simulink model "EReg_Tank_Drain"  (R2025b)
settings: Solver=ode1  StartTime=0.0  StopTime=12  FixedStep=0.001  RelTol=1e-3
values from neighbouring files (symbols this model uses):
  A_3 = 13.27e-6    (= 1.327e-05)    [EReg_N2O_Simulink_Init.m]    (also in EReg_Tank_Drain_Init.m = 6e-05)
  Cd_3 = 0.6    [EReg_N2O_Simulink_Init.m]    (also in EReg_Tank_Drain_Init.m = 0.7)
  Feedforward = 0    [EReg_N2O_Simulink_Init.m]    (also in EReg_Tank_Drain_Init.m)
  hL_LUT = n2o_tab.h_L    [EReg_N2O_Simulink_Init.m]
  K_D = 3    [EReg_N2O_Simulink_Init.m]    (also in EReg_Tank_Drain_Init.m = 8; EReg_Tank_Drain_N2O_Sim.m = params.K_D)
  K_I = 15    [EReg_N2O_Simulink_Init.m]    (also in EReg_Tank_Drain_Init.m = 17; EReg_Tank_Drain_N2O_Sim.m = params.K_I)
  K_P = 20    [EReg_N2O_Simulink_Init.m]    (also in EReg_Tank_Drain_Init.m = 16; EReg_Tank_Drain_N2O_Sim.m = params.K_P)
  Kv_1_max = 1.5    [EReg_N2O_Simulink_Init.m]    (also in EReg_Tank_Drain_Init.m = 1; EReg_Tank_Drain_N2O_Sim.m = params.Kv_1_max)
  Kv_2 = 1    [EReg_Tank_Drain_Init.m]
  m_1_0 = rho_1_0 * V_1    (= 2.35097796073)    [EReg_N2O_Simulink_Init.m]    (also in EReg_Tank_Drain_Init.m = 2.2972972973; EReg_Tank_Drain_N2O_Sim.m = params.m_1_0)
  m_N2_ull_0 = rho_N2_init * V_ull_init    [EReg_N2O_Simulink_Init.m]
  m_N2O_liq_0 = 12    [EReg_N2O_Simulink_Init.m]
  P_1_0 = 300e5    (= 30000000)    [EReg_N2O_Simulink_Init.m]    (also in EReg_Tank_Drain_Init.m; EReg_Tank_Drain_N2O_Sim.m = params.P_1_0)
  P_atm = 25e5    (= 2500000)    [EReg_N2O_Simulink_Init.m]    (also in EReg_Tank_Drain_Init.m = 0; EReg_Tank_Drain_N2O_Sim.m = params.P_atm)
  P_sat_LUT = n2o_tab.P    [EReg_N2O_Simulink_Init.m]
  R_N2 = 296    [EReg_N2O_Simulink_Init.m]    (also in EReg_Tank_Drain_Init.m; EReg_Tank_Drain_N2O_Sim.m = params.R_N2)
  rho_1_0 = P_1_0 / (R_N2 * T_0_N2)    (= 345.732053049)    [EReg_N2O_Simulink_Init.m]    (also in EReg_Tank_Drain_Init.m = 337.837837838; EReg_Tank_Drain_N2O_Sim.m = m_1_0 / V_1)
  rhoL_LUT = n2o_tab.rho_L    [EReg_N2O_Simulink_Init.m]
  rhoV_LUT = n2o_tab.rho_V    [EReg_N2O_Simulink_Init.m]
  servo_off_setpoint = ones(1, Num_Steps)    [EReg_N2O_Simulink_Init.m]    (also in EReg_Tank_Drain_Init.m = zeros(1, Num_Steps))
  T_1_0 = T_0_N2    (= 293.15)    [EReg_N2O_Simulink_Init.m]    (also in EReg_Tank_Drain_N2O_Sim.m = P_1_0 / (rho_1_0 * R_N2))
  T_N2O_0 = T_0_N2    (= 293.15)    [EReg_N2O_Simulink_Init.m]
  T_sat_LUT = n2o_tab.T    [EReg_N2O_Simulink_Init.m]
  time = linspace(0, Sim_Duration, Num_Steps)    [EReg_N2O_Simulink_Init.m]    (also in EReg_Tank_Drain_Init.m; EReg_Tank_Drain_N2O_Sim.m = (0 : dt : t_end)')
  U_N2O_0 = m_N2O_liq_0 * uL_init + m_N2O_vap_init * uV_init    [EReg_N2O_Simulink_Init.m]
  uL_LUT = n2o_tab.u_L    [EReg_N2O_Simulink_Init.m]
  uV_LUT = n2o_tab.u_V    [EReg_N2O_Simulink_Init.m]
  V_1 = 6.8e-3    (= 0.0068)    [EReg_N2O_Simulink_Init.m]    (also in EReg_Tank_Drain_Init.m; EReg_Tank_Drain_N2O_Sim.m = params.V_1)
  V_2 = 30e-3    (= 0.03)    [EReg_N2O_Simulink_Init.m]    (also in EReg_Tank_Drain_Init.m = 0.025; EReg_Tank_Drain_N2O_Sim.m = params.V_2)
libraries: simulink x4, slpidlib x2
settings Model: Creator=marti  LastModifiedBy=Aziz
settings OptimizationCC: ReuseModelBlockBuffer=off
settings RTWCC: GPUComputeCapability=3.5

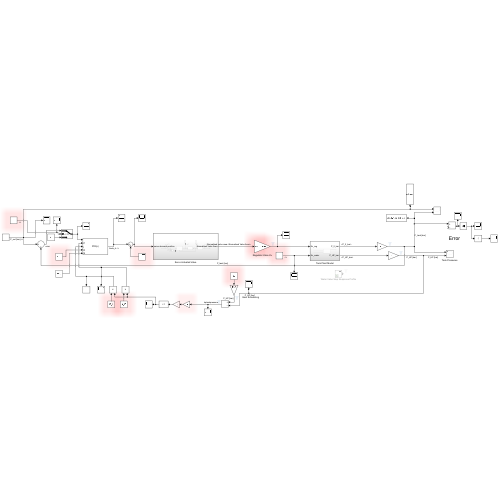
[thumbnail: Simulink's stored preview of the top-level diagram]
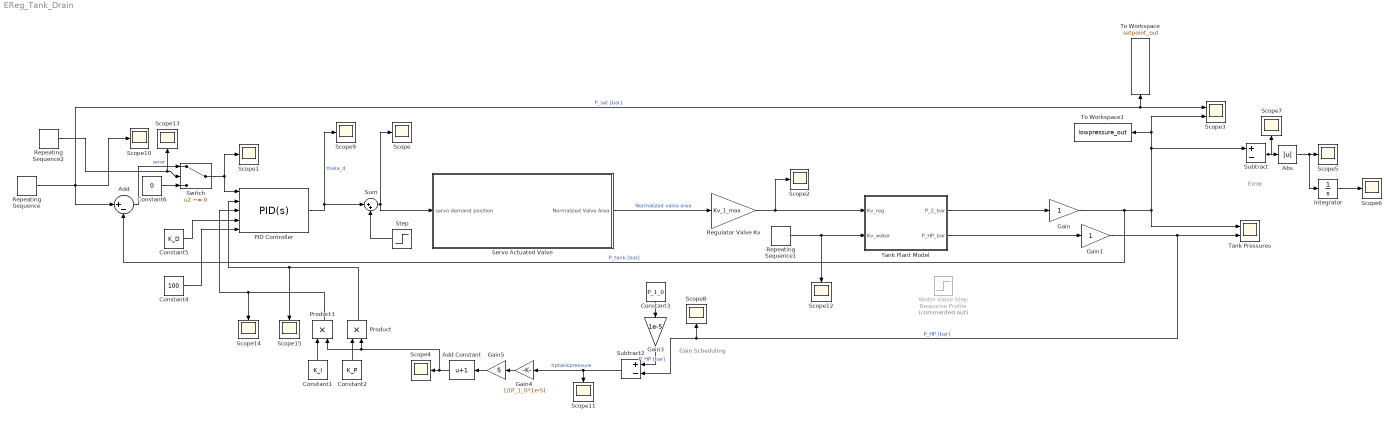
== system EReg_Tank_Drain ==
  note: Gain Scheduling
  note: Error
  Abs : Abs  SaturateOnIntegerOverflow=off
  Add : Sum  Inputs=|+-
  Add Constant : Bias  Bias=1  SaturateOnIntegerOverflow=off
  Constant1 : Constant  Value=K_I
  Constant2 : Constant  Value=K_P
  Constant3 : Constant  Value=P_1_0
  Constant4 : Constant  Value=100
  Constant5 : Constant  Value=K_D
  Constant6 : Constant  Value=0
  Gain : Gain
  Gain1 : Gain
  Gain3 : Gain  Gain=1e-5
  Gain4 : Gain  Gain=1/(P_1_0*1e-5)
  Gain5 : Gain  Gain=5
  Integrator : Integrator
  PID Controller : slpidlib/PID Controller  Controller=PID  Form=Parallel  TimeDomain=Continuous-time  UseExternalTs=off  SampleTime=-1  IntegratorMethod=Forward Euler  FilterMethod=Forward Euler  ControllerParametersSource=external  P=1.5  I=3  UseKiTs=off  D=0  UseExternalDerivativeSource=off  N=100  UseFilter=on  TunerSelectOption=Transfer Function Based (PID Tuner App)  InitialConditionSource=internal  InitialConditionForIntegrator=0  InitialConditionForFilter=0  DifferentiatorICPrevScaledInput=0  ExternalReset=none  TrackingMode=off  Kt=1  LimitOutput=off  SatLimitsSource=internal  UpperSaturationLimit=180  LowerSaturationLimit=0  LinearizeAsGain=on  AntiWindupMode=clamping  Kb=1  LimitIntegrator=on  UpperIntegratorSaturationLimit=20  LowerIntegratorSaturationLimit=-20  POutMin=[]  POutMax=[]  IOutMin=[]  IOutMax=[]  DOutMin=[]  DOutMax=[]  NOutMin=[]  NOutMax=[]  SumOutMin=[]  SumOutMax=[]  SaturationOutMin=[]  SaturationOutMax=[]  PParamMin=[]  PParamMax=[]  IParamMin=[]  IParamMax=[]  DParamMin=[]  DParamMax=[]  NParamMin=[]  NParamMax=[]  KbParamMin=[]  KbParamMax=[]  KtParamMin=[]  KtParamMax=[]  KbOutMin=[]  KbOutMax=[]  KtOutMin=[]  KtOutMax=[]  IntegratorOutMin=[]  IntegratorOutMax=[]  FilterOutMin=[]  FilterOutMax=[]  SumI1OutMin=[]  SumI1OutMax=[]  SumI2OutMin=[]  SumI2OutMax=[]  SumI3OutMin=[]  SumI3OutMax=[]  SumI4OutMin=[]  SumI4OutMax=[]  SumDOutMin=[]  SumDOutMax=[]  DifferentiatorOutMin=[]  DifferentiatorOutMax=[]  FilterDiffOutCoefMin=[]  FilterDiffOutCoefMax=[]  ReciprocalOutMin=[]  ReciprocalOutMax=[]  SumDenOutMin=[]  SumDenOutMax=[]  SumNumOutMin=[]  SumNumOutMax=[]  DivideOutMin=[]  DivideOutMax=[]  UdiffTsProdOutMin=[]  UdiffTsProdOutMax=[]  NTsProdOutMin=[]  NTsProdOutMax=[]  UintegralTsProdOutMin=[]  UintegralTsProdOutMax=[]  UngainTsProdOutMin=[]  UngainTsProdOutMax=[]  ClampingZeroOutDataTypeStr=Inherit: Inherit via back propagation  ClampingZeroOutMin=[]  ClampingZeroOutMax=[]  FilterDenConstantOutDataTypeStr=Inherit: Inherit via back propagation  FilterDenConstantOutMin=[]  FilterDenConstantOutMax=[]  PCopyOutDataTypeStr=Inherit: Inherit via back propagation  PCopyOutMin=[]  PCopyOutMax=[]  NCopyOutDataTypeStr=Inherit: Inherit via back propagation  NCopyOutMin=[]  NCopyOutMax=[]  IntegratorContinuousStateAttributes=''  IntegratorStateMustResolveToSignalObject=off  IntegratorRTWStateStorageClass=Auto  FilterContinuousStateAttributes=''  FilterStateMustResolveToSignalObject=off  FilterRTWStateStorageClass=Auto  ParallelPVariant=ExternalParameters  IdealPVariant=Disabled  IVariant=ExternalParameters  DVariant=ExternalParameters  IntegratorVariant=Continuous  SatVariant=Disabled  AWVariant=Passthrough  PCopyVariant=Disabled  TRVariant=Disabled  FdbkBlocksVariant=Forward  IdealPFdbkVariant=Disabled  SatFdbkVariant=Disabled  DerivativeFilterVariant=ContFilter  NVariant=ExternalParameters  NCopyVariant=Disabled  FilterICVariant=InternalICsFilter  IntegratorICVariant=InternalICs  ExternalResetVariant=Disabled  TRSumVariant=Passthrough  SumFdbkVariant=Disabled  SumVariant=Sum_PID  TsampFilterVariant=InternalTs  TsampNgainVariant=Passthrough  TsampIntegralVariant=Disabled_SignalSpec  ExternalSaturationOutDataTypeStr=Inherit: Same as second input  DerivativeSourceVariant=ErrorSignal  PreIntVariant=InternalPreInt
  Product : Product
  Product1 : Product
  Regulator Valve Kv : Gain  Gain=Kv_1_max
  Repeating Sequence : simulink/Sources/Repeating Sequence  rep_seq_t=time  rep_seq_y=setpoint
  Repeating Sequence1 : simulink/Sources/Repeating Sequence  rep_seq_t=time  rep_seq_y=run_valve_setpoint
  Repeating Sequence2 : simulink/Sources/Repeating Sequence  rep_seq_t=time  rep_seq_y=run_valve_setpoint
  Scope{,1..2,4..15} (15 alike) : Scope
      Scope settings: ActiveDisplayYMinimum=-1688.77171  ActiveDisplayYMaximum=357.47639  DataLoggingVariableName=ScopeData7
      Scope1 settings: ActiveDisplayYMinimum=-2.28363  ActiveDisplayYMaximum=0.62203
      Scope10 settings: ActiveDisplayYMinimum=51.3375  ActiveDisplayYMaximum=67.98472  DataLoggingVariableName=ScopeData2
      Scope11 settings: ActiveDisplayYMinimum=-7.98984  ActiveDisplayYMaximum=71.90855
      Scope12 settings: ActiveDisplayYMinimum=-0.125  ActiveDisplayYMaximum=1.125  DataLoggingVariableName=ScopeData2
      Scope13 settings: ActiveDisplayYMinimum=-0.125  ActiveDisplayYMaximum=1.125  DataLoggingVariableName=ScopeData3
      Scope14 settings: ActiveDisplayYMinimum=5.20102  ActiveDisplayYMaximum=13.19086
      Scope15 settings: ActiveDisplayYMinimum=13.00254  ActiveDisplayYMaximum=32.97714  DataLoggingVariableName=ScopeData2
      Scope2 settings: ActiveDisplayYMinimum=-0.0196  ActiveDisplayYMaximum=0.17636
      Scope4 settings: ActiveDisplayYMinimum=0.86684  ActiveDisplayYMaximum=2.19848
      Scope5 settings: ActiveDisplayYMinimum=-0.46907  ActiveDisplayYMaximum=4.2216
      Scope6 settings: ActiveDisplayYMinimum=-42.4732  ActiveDisplayYMaximum=382.25884  DataLoggingVariableName=ScopeData2
      Scope7 settings: ActiveDisplayYMinimum=-4.72126  ActiveDisplayYMaximum=4.96726  DataLoggingVariableName=ScopeData3
      Scope8 settings: ActiveDisplayYMinimum=229.43787  ActiveDisplayYMaximum=307.84024  DataLoggingVariableName=ScopeData4
      Scope9 settings: ActiveDisplayYMinimum=-1660.50954  ActiveDisplayYMaximum=362.9195  DataLoggingVariableName=ScopeData5
  Scope3 : Scope  NumInputPorts=2
      settings: ActiveDisplayYMinimum=51.75312  ActiveDisplayYMaximum=64.23854
  Servo Actuated Valve : Subsystem
  Step : Step  After=Feedforward  SampleTime=0
  Subtract : Sum  Inputs=+-
  Subtract2 : Sum  Inputs=+-
  Sum : Sum  Inputs=|++
  Switch : Switch  Criteria=u2 ~= 0  SaturateOnIntegerOverflow=off  InputSameDT=off
  Tank Plant Model : Subsystem
  Tank Pressures : Scope  NumInputPorts=2
      settings: ActiveDisplayYMinimum=22.037093774647268  ActiveDisplayYMaximum=330.88476735837253
  To Workspace : ToWorkspace  VariableName=setpoint_out  SaveFormat=Timeseries  SampleTime=-1
  To Workspace1 : ToWorkspace  VariableName=lowpressure_out  SaveFormat=Timeseries  SampleTime=-1
  Water Valve Step Response Profile : Step  Commented=on  After=Kv_2  SampleTime=0
  wires:
  Tank Plant Model/1(P_2_bar) -> Gain/1
  Tank Plant Model/2(P_HP_bar) -> Gain1/1
  Servo Actuated Valve/1(Normalized Valve Area) -> Regulator Valve Kv/1  "Normalized valve area"
  Gain/1 -> Subtract/1, Scope3/2, To Workspace1/1, Tank Pressures/1, Add/2  "P_tank [bar]"
  Gain1/1 -> Subtract2/2, Scope8/1, Tank Pressures/2  "P_HP [bar]"
  Regulator Valve Kv/1 -> Tank Plant Model/1(Kv_reg), Scope2/1
  PID Controller/1 -> Scope9/1, Sum/1  "theta_d"
  Sum/1 -> Scope/1, Servo Actuated Valve/1(servo demand position)
  Subtract/1 -> Scope7/1, Abs/1
  Abs/1 -> Integrator/1, Scope5/1
  Integrator/1 -> Scope6/1
  Subtract2/1 -> Scope11/1, Gain4/1  "hptankpressure"
  Constant3/1 -> Gain3/1
  Gain3/1 -> Subtract2/1  "P_HP [bar]"
  Add Constant/1 -> Product1/2, Product/2, Scope4/1
  Constant2/1 -> Product/1
  Constant1/1 -> Product1/1
  Product/1 -> Scope15/1, PID Controller/2
  Product1/1 -> PID Controller/3, Scope14/1
  Step/1 -> Sum/2
  Gain4/1 -> Gain5/1
  Gain5/1 -> Add Constant/1
  Constant4/1 -> PID Controller/5
  Constant5/1 -> PID Controller/4
  Repeating Sequence1/1 -> Scope12/1, Tank Plant Model/2(Kv_water)
  Switch/1 -> Scope1/1, PID Controller/1
  Constant6/1 -> Switch/3
  Add/1 -> Switch/1  "error"
  Repeating Sequence2/1 -> Switch/2, Scope13/1
  Repeating Sequence/1 -> To Workspace/1, Scope3/1, Scope10/1, Add/1  "P_set [bar]"

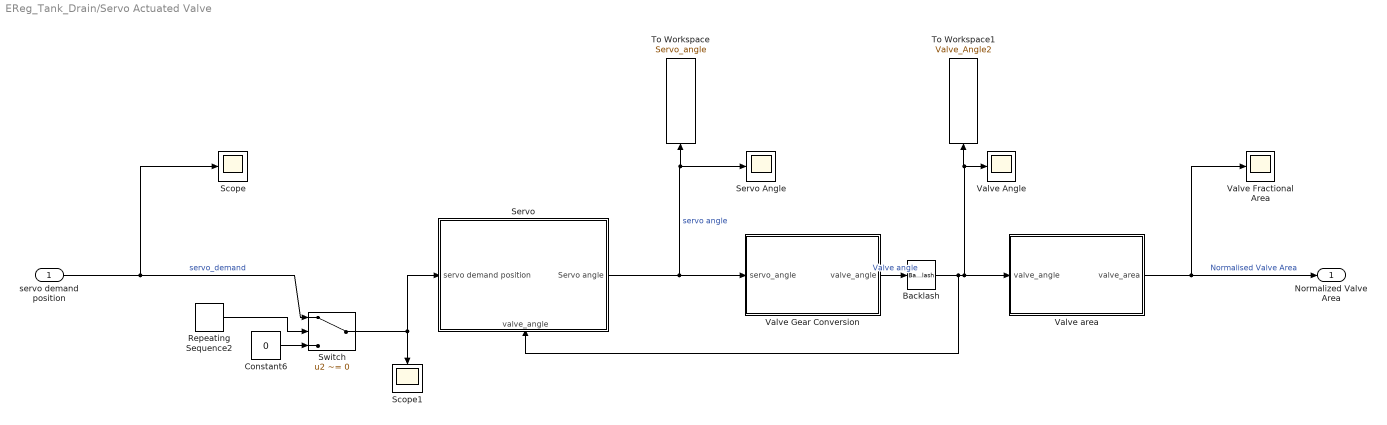
== system EReg_Tank_Drain/Servo Actuated Valve ==
  servo demand position : Inport
  " Valve Gear Conversion" : MATLAB Function  TreatAsAtomicUnit=on
  " Valve area" : MATLAB Function  TreatAsAtomicUnit=on
  Backlash : Backlash  BacklashWidth=0.5  InitialOutput=0.5
  Constant6 : Constant  Value=0
  Repeating Sequence2 : simulink/Sources/Repeating Sequence  rep_seq_t=time(:)  rep_seq_y=servo_off_setpoint(:)
  Scope : Scope
      settings: ActiveDisplayYMinimum=-1660.50954  ActiveDisplayYMaximum=362.9195  DataLoggingVariableName=ScopeData3
  Scope1 : Scope
      settings: ActiveDisplayYMinimum=-1660.50954  ActiveDisplayYMaximum=362.9195  DataLoggingVariableName=ScopeData3
  Servo : Subsystem
      settings: PortSchema="{\"entries\":[{\"content\":{\"sides\":[{\"content\":{\"connectorIds\":[\"In1\"]},\"type\":\"ConnectorPlacement.EquallySpacedRectSide\",\"uuid\":\"80cc8390-5c54-44fd-a47c-7e7786ca55cb\"},{\"content\":{\"connectorIds\":[\"Out1\"],\"side\":\"RIGHT\"},\"type\":\"ConnectorPlacement.EquallySpacedRectSide\",\"uuid\":\"1eac09ca-847a-4c9b-93fa-12e39acf6b4a\"},{\"content\":{\"side\":\"TOP\"},\"type\":\"ConnectorPlacement.EquallySpacedRectSide\",\"uuid\":\"448ec877-4708-4b6f-bd0d-b7e31e141685\"},{\"content\":{\"connectorIds\":[\"In2\"],\"side\":\"BOTTOM\"},\"type\":\"ConnectorPlacement.EquallySpacedRectSide\",\"uuid\":\"b9bb9fb8-2143-4f55-8173-037b619887c5\"}]},\"type\":\"ConnectorPlacement.EquallySpacedConnector\",\"uuid\":\"bf70c898-a427-4eb9-a0e2-218e58098715\"}],\"packageUris\":[\"http://schema.mathworks.com/mf0/Connector/R2020b\"],\"version\":\"1.0\"}"
  Servo Angle : Scope
      settings: ActiveDisplayYMinimum=-2.83907  ActiveDisplayYMaximum=21.23036  DataLoggingVariableName=Servo_Angle  DataLoggingSaveFormat=Array
  Switch : Switch  Criteria=u2 ~= 0  SaturateOnIntegerOverflow=off  InputSameDT=off
  To Workspace : ToWorkspace  VariableName=Servo_angle  SampleTime=-1
      settings: Save2DSignal=2-D array (concatenate along first dimension)
  To Workspace1 : ToWorkspace  VariableName=Valve_Angle2  SampleTime=-1
      settings: Save2DSignal=2-D array (concatenate along first dimension)
  Valve Angle : Scope
      settings: ActiveDisplayYMinimum=-1.35754  ActiveDisplayYMaximum=12.17595  DataLoggingVariableName=Valve_Angle  DataLoggingSaveFormat=Array
  Valve Fractional Area : Scope
      settings: ActiveDisplayYMinimum=-0.0196  ActiveDisplayYMaximum=0.17636  DataLoggingVariableName=ScopeData8
  Normalized Valve Area : Outport
  wires:
  " Valve area"/1(valve_area) -> Normalized Valve Area/1, Valve Fractional Area/1  "Normalised Valve Area"
  " Valve Gear Conversion"/1(valve_angle) -> Backlash/1  "Valve angle"
  servo demand position/1 -> Scope/1, Switch/1  "servo_demand"
  Servo/1(Servo angle) -> " Valve Gear Conversion"/1(servo_angle), To Workspace/1, Servo Angle/1  "servo angle"
  Repeating Sequence2/1 -> Switch/2
  Constant6/1 -> Switch/3
  Switch/1 -> Servo/1(servo demand position), Scope1/1
  Backlash/1 -> " Valve area"/1(valve_angle), To Workspace1/1, Valve Angle/1, Servo/2(valve_angle)

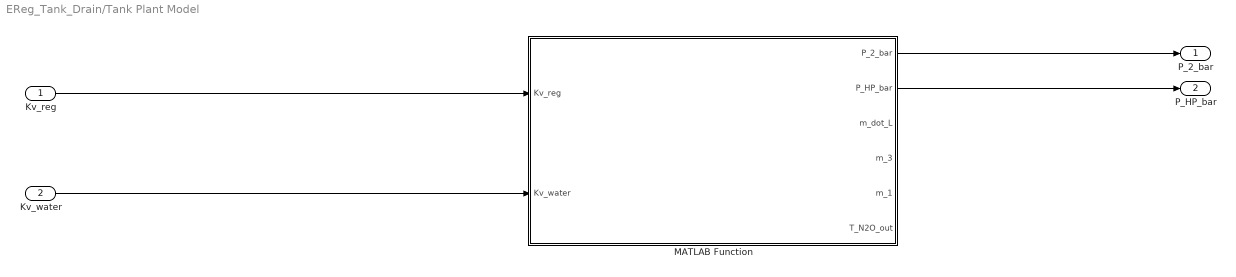
== system EReg_Tank_Drain/Tank Plant Model ==
  Kv_reg : Inport
  Kv_water : Inport  Port=2
  MATLAB Function : MATLAB Function  TreatAsAtomicUnit=on
  P_2_bar : Outport
  P_HP_bar : Outport  Port=2
  wires:
  Kv_reg/1 -> MATLAB Function/1(Kv_reg)
  Kv_water/1 -> MATLAB Function/2(Kv_water)
  MATLAB Function/1(P_2_bar) -> P_2_bar/1
  MATLAB Function/2(P_HP_bar) -> P_HP_bar/1

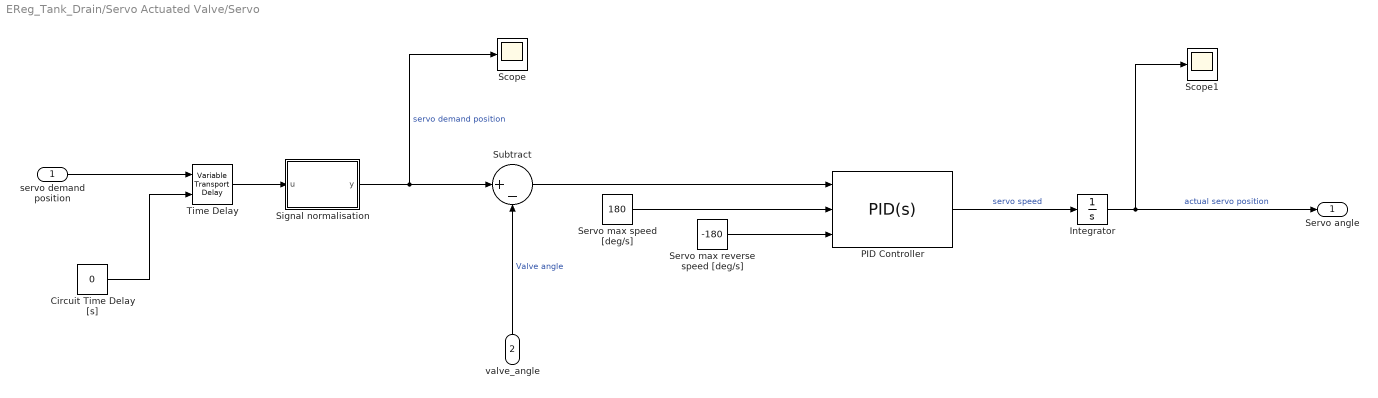
== system EReg_Tank_Drain/Servo Actuated Valve/Servo ==
  servo demand position : Inport
  valve_angle : Inport  Port=2
  Circuit Time Delay [s] : Constant  Value=0
  Integrator : Integrator
  PID Controller : slpidlib/PID Controller  Controller=PID  Form=Parallel  TimeDomain=Continuous-time  UseExternalTs=off  SampleTime=-1  IntegratorMethod=Forward Euler  FilterMethod=Forward Euler  ControllerParametersSource=internal  P=3  I=2  UseKiTs=off  D=0  UseExternalDerivativeSource=off  N=100  UseFilter=on  TunerSelectOption=Transfer Function Based (PID Tuner App)  InitialConditionSource=internal  InitialConditionForIntegrator=0  InitialConditionForFilter=0  DifferentiatorICPrevScaledInput=0  ExternalReset=none  TrackingMode=off  Kt=1  LimitOutput=on  SatLimitsSource=external  UpperSaturationLimit=inf  LowerSaturationLimit=-inf  LinearizeAsGain=on  AntiWindupMode=none  Kb=1  LimitIntegrator=off  UpperIntegratorSaturationLimit=inf  LowerIntegratorSaturationLimit=-inf  POutMin=[]  POutMax=[]  IOutMin=[]  IOutMax=[]  DOutMin=[]  DOutMax=[]  NOutMin=[]  NOutMax=[]  SumOutMin=[]  SumOutMax=[]  SaturationOutMin=[]  SaturationOutMax=[]  PParamMin=[]  PParamMax=[]  IParamMin=[]  IParamMax=[]  DParamMin=[]  DParamMax=[]  NParamMin=[]  NParamMax=[]  KbParamMin=[]  KbParamMax=[]  KtParamMin=[]  KtParamMax=[]  KbOutMin=[]  KbOutMax=[]  KtOutMin=[]  KtOutMax=[]  IntegratorOutMin=[]  IntegratorOutMax=[]  FilterOutMin=[]  FilterOutMax=[]  SumI1OutMin=[]  SumI1OutMax=[]  SumI2OutMin=[]  SumI2OutMax=[]  SumI3OutMin=[]  SumI3OutMax=[]  SumI4OutMin=[]  SumI4OutMax=[]  SumDOutMin=[]  SumDOutMax=[]  DifferentiatorOutMin=[]  DifferentiatorOutMax=[]  FilterDiffOutCoefMin=[]  FilterDiffOutCoefMax=[]  ReciprocalOutMin=[]  ReciprocalOutMax=[]  SumDenOutMin=[]  SumDenOutMax=[]  SumNumOutMin=[]  SumNumOutMax=[]  DivideOutMin=[]  DivideOutMax=[]  UdiffTsProdOutMin=[]  UdiffTsProdOutMax=[]  NTsProdOutMin=[]  NTsProdOutMax=[]  UintegralTsProdOutMin=[]  UintegralTsProdOutMax=[]  UngainTsProdOutMin=[]  UngainTsProdOutMax=[]  ClampingZeroOutDataTypeStr=Inherit: Inherit via back propagation  ClampingZeroOutMin=[]  ClampingZeroOutMax=[]  FilterDenConstantOutDataTypeStr=Inherit: Inherit via back propagation  FilterDenConstantOutMin=[]  FilterDenConstantOutMax=[]  PCopyOutDataTypeStr=Inherit: Inherit via back propagation  PCopyOutMin=[]  PCopyOutMax=[]  NCopyOutDataTypeStr=Inherit: Inherit via back propagation  NCopyOutMin=[]  NCopyOutMax=[]  IntegratorContinuousStateAttributes=''  IntegratorStateMustResolveToSignalObject=off  IntegratorRTWStateStorageClass=Auto  FilterContinuousStateAttributes=''  FilterStateMustResolveToSignalObject=off  FilterRTWStateStorageClass=Auto  ParallelPVariant=InternalParameters  IdealPVariant=Disabled  IVariant=InternalParameters  DVariant=InternalParameters  IntegratorVariant=Continuous  SatVariant=External  AWVariant=Passthrough  PCopyVariant=Disabled  TRVariant=Disabled  FdbkBlocksVariant=Forward  IdealPFdbkVariant=Disabled  SatFdbkVariant=Disabled  DerivativeFilterVariant=ContFilter  NVariant=InternalParameters  NCopyVariant=Disabled  FilterICVariant=InternalICsFilter  IntegratorICVariant=InternalICs  ExternalResetVariant=Disabled  TRSumVariant=Passthrough  SumFdbkVariant=Disabled  SumVariant=Sum_PID  TsampFilterVariant=InternalTs  TsampNgainVariant=Passthrough  TsampIntegralVariant=Disabled_SignalSpec  ExternalSaturationOutDataTypeStr=Inherit: Same as second input  DerivativeSourceVariant=ErrorSignal  PreIntVariant=InternalPreInt
  Scope : Scope
      settings: ActiveDisplayYMinimum=-20.07207  ActiveDisplayYMaximum=180.64867
  Scope1 : Scope
      settings: ActiveDisplayYMinimum=-2.83907  ActiveDisplayYMaximum=21.23036  DataLoggingVariableName=ScopeData2
  Servo max reverse speed [deg/s] : Constant  Value=-180
  Servo max speed [deg/s] : Constant  Value=180
  Signal normalisation : MATLAB Function  TreatAsAtomicUnit=on
  Subtract : Sum  Inputs=|+-
  Time Delay : VariableTransportDelay  MaximumDelay=10  MaximumPoints=6000  ZeroDelay=on
  Servo angle : Outport
  wires:
  Servo max reverse speed [deg/s]/1 -> PID Controller/3
  Servo max speed [deg/s]/1 -> PID Controller/2
  PID Controller/1 -> Integrator/1  "servo speed"
  Integrator/1 -> Scope1/1, Servo angle/1  "actual servo position"
  Subtract/1 -> PID Controller/1
  Signal normalisation/1(y) -> Scope/1, Subtract/1  "servo demand position"
  servo demand position/1 -> Time Delay/1
  Time Delay/1 -> Signal normalisation/1(u)
  Circuit Time Delay [s]/1 -> Time Delay/2
  valve_angle/1 -> Subtract/2  "Valve angle"

== matlab function EReg_Tank_Drain/Tank Plant Model/MATLAB Function ==
  settings: updateMethod=DISCRETE
  data: Kv_reg input; P_2_bar output; Kv_water input; P_HP_bar output; m_dot_L output; m_3 output; m_1 output; T_N2O_out output; V_1 parameter; V_2 parameter; A_3 parameter; Cd_3 parameter; R_N2 parameter; P_atm parameter; hL_LUT parameter; uV_LUT parameter; uL_LUT parameter; rhoV_LUT parameter; rhoL_LUT parameter; P_sat_LUT parameter; T_sat_LUT parameter; T_1_0 parameter; rho_1_0 parameter; P_1_0 parameter; U_N2O_0 parameter; T_N2O_0 parameter; m_N2_ull_0 parameter; m_1_0 parameter; m_N2O_liq_0 parameter
function [P_2_bar, P_HP_bar, m_dot_L, m_3, m_1, T_N2O_out] = N2O_Tank_Plant(Kv_reg, Kv_water, ...
    V_1, V_2, A_3, Cd_3, R_N2, P_atm, ...
hL_LUT, ...
uV_LUT, uL_LUT, rhoV_LUT, rhoL_LUT, P_sat_LUT, T_sat_LUT, T_1_0, rho_1_0, P_1_0, U_N2O_0, T_N2O_0, m_N2_ull_0, m_1_0, m_N2O_liq_0)
%#codegen
% N2O_Tank_Plant - Two-phase N2O tank plant for Simulink MATLAB Function block
%
% This function computes one time step of the N2O tank thermodynamics.
% It is designed to be called from a MATLAB Function block in Simulink.
%
% INPUTS (from Simulink signals):
%   Kv_reg      - Regulator valve Kv (from controller via servo model) [normalised 0-1]
%   Kv_water    - Water/run valve Kv (0 = closed, 1 = open)
%
% INPUTS (from workspace/parameters):
%   V_1, V_2    - Tank volumes [m^3]
%   A_3, Cd_3   - Injector area and discharge coefficient
%   R_N2        - N2 gas constant [J/kgK]
%   P_atm       - Downstream/chamber pressure [Pa]
%   T_sat_LUT, P_sat_LUT, rhoL_LUT, rhoV_LUT, uL_LUT, uV_LUT, hL_LUT
%               - N2O saturation LUT vectors (indexed by row, same length)
%
% INPUTS (persistent state, initialised from workspace):
%   m_1_0, m_N2O_liq_0, m_N2_ull_0, T_N2O_0, U_N2O_0, P_1_0, rho_1_0, T_1_0
%               - Initial conditions
%
% OUTPUTS (to Simulink):
%   P_2_bar     - Run tank total pressure [bar]
%   P_HP_bar    - HP N2 tank pressure [bar]
%   m_dot_L     - Liquid N2O mass flow through injector [kg/s]
%   m_3         - N2O liquid mass remaining [kg]
%   m_1         - N2 mass remaining in HP tank [kg]
%   T_N2O_out   - N2O liquid temperature [K]

% ---- Persistent State Variables ----
persistent m1 m_N2O_liq m_N2O_vap m_N2_ull T_N2O U_N2O rho1 T1 m_N2O_total initialised

if isempty(initialised) 
    m1          = m_1_0;
    m_N2O_liq   = m_N2O_liq_0;
    T_N2O       = T_N2O_0;
    U_N2O       = U_N2O_0;
    rho1        = rho_1_0;
    T1          = T_1_0;
    m_N2_ull    = m_N2_ull_0;

    % Compute initial vapour mass
    rhoV_init   = interp1_lut(T_sat_LUT, rhoV_LUT, T_N2O);
    rhoL_init   = interp1_lut(T_sat_LUT, rhoL_LUT, T_N2O);
    V_liq_init  = m_N2O_liq / rhoL_init;
    V_ull_init  = V_2 - V_liq_init;
    m_N2O_vap   = rhoV_init * max(V_ull_init, 1e-6);
    m_N2O_total = m_N2O_liq + m_N2O_vap;

    initialised = 1;
end

% ---- Sample Time ----
dt = 0.001;  % Must match Simulink fixed-step solver (1 ms)

% ---- Polytropic N2 index ----
n_poly = 1.3;
gamma_N2 = 1.4;

% ---- Clamp T_N2O to LUT range ----
T_min = T_sat_LUT(1)   + 0.5;
T_max = T_sat_LUT(end) - 2.0;
T_N2O = max(T_min, min(T_max, T_N2O));

% ======== HP TANK (N2 source) ========
rho1 = m1 / V_1;
T1   = T_1_0 * (rho1 / rho_1_0)^(n_poly - 1);
T1   = max(T1, 200);
P_1  = rho1 * R_N2 * T1;

% ======== RUN TANK (N2O + N2 ullage) ========
P_vap = interp1_lut(T_sat_LUT, P_sat_LUT, T_N2O);
rho_L = interp1_lut(T_sat_LUT, rhoL_LUT, T_N2O);
rho_V = interp1_lut(T_sat_LUT, rhoV_LUT, T_N2O);
u_L   = interp1_lut(T_sat_LUT, uL_LUT,   T_N2O);
u_V   = interp1_lut(T_sat_LUT, uV_LUT,   T_N2O);
h_L   = interp1_lut(T_sat_LUT, hL_LUT,   T_N2O);

% Volumes
if m_N2O_liq > 0.001
    V_liq = m_N2O_liq / rho_L;
    V_ull = max(V_2 - V_liq, 1e-6);
else
    V_liq = 0;
    V_ull = V_2;
    m_N2O_liq = 0;
end

% Partial pressures (Dalton's Law)
P_N2_partial = (m_N2_ull * R_N2 * T_N2O) / V_ull;
P_2 = P_N2_partial + P_vap;

% ======== FLOW CALCULATIONS ========

% --- Regulator: N2 from HP -> Run tank ullage ---
Kv_max_area = 1.5;  % Must match init file Kv_1_max
A_valve_max = 2.4e-5 * Kv_max_area;
A_reg_eff   = A_valve_max * Kv_reg;  % Kv_reg is 0-1 normalised

if P_1 > P_2 && A_reg_eff > 0
    m_dot_reg = gas_flow(P_1, P_2, T1, R_N2, gamma_N2, A_reg_eff);
else
    m_dot_reg = 0;
end

% --- Injector: Liquid N2O from tank -> chamber ---
if Kv_water > 0.5 && m_N2O_liq > 0.001
    dP_inj = P_2 - P_atm;
    if dP_inj > 0
        m_dot_inj = Cd_3 * A_3 * sqrt(2 * rho_L * dP_inj);
    else
        m_dot_inj = 0;
    end
else
    m_dot_inj = 0;
end

% ======== STATE UPDATE (Forward Euler) ========

% Mass updates
m1        = max(0, m1 - m_dot_reg * dt);
m_N2_ull  = m_N2_ull + m_dot_reg * dt;
m_N2O_liq = max(0, m_N2O_liq - m_dot_inj * dt);
m_N2O_total = m_N2O_liq + m_N2O_vap;

% Energy balance
dU_out      = m_dot_inj * h_L * dt;
Cp_N2       = R_N2 * gamma_N2 / (gamma_N2 - 1);
dU_N2_heat  = m_dot_reg * Cp_N2 * (T1 - T_N2O) * dt * 0.1;
U_N2O       = U_N2O - dU_out + dU_N2_heat;

% Solve for new temperature (simplified Newton — 5 iterations max)
if m_N2O_liq > 0.001
    T_N2O = solve_T(T_N2O, U_N2O, m_N2O_total, V_2, ...
                     T_sat_LUT, rhoL_LUT, rhoV_LUT, uL_LUT, uV_LUT, T_min, T_max);

    % Recompute phase split
    rho_L_n = interp1_lut(T_sat_LUT, rhoL_LUT, T_N2O);
    rho_V_n = interp1_lut(T_sat_LUT, rhoV_LUT, T_N2O);
    denom = 1 - rho_V_n / rho_L_n;
    if abs(denom) > 1e-9
        m_N2O_liq = max(0, (m_N2O_total - rho_V_n * V_2) / denom);
    end
    m_N2O_vap = max(0, m_N2O_total - m_N2O_liq);
end

% ======== OUTPUTS ========
P_2_bar   = P_2 / 1e5;
P_HP_bar  = P_1 / 1e5;
m_dot_L   = m_dot_inj;
m_3       = m_N2O_liq;
m_1       = m1;
T_N2O_out = T_N2O;

end

% ======== LOCAL FUNCTIONS ========

function y = interp1_lut(x_vec, y_vec, x_q)
%#codegen
% Linear interpolation with clamping (codegen compatible)
    n = length(x_vec);
    if x_q <= x_vec(1)
        y = y_vec(1);
        return;
    end
    if x_q >= x_vec(n)
        y = y_vec(n);
        return;
    end
    % Binary search
    lo = 1; hi = n;
    while hi - lo > 1
        mid = floor((lo + hi) / 2);
        if x_vec(mid) <= x_q
            lo = mid;
        else
            hi = mid;
        end
    end
    frac = (x_q - x_vec(lo)) / (x_vec(hi) - x_vec(lo));
    y = y_vec(lo) + frac * (y_vec(hi) - y_vec(lo));
end

function m_dot = gas_flow(P_up, P_down, T_up, R, gamma, Area)
%#codegen
    PR = P_down / P_up;
    PR_crit = (2/(gamma+1))^(gamma/(gamma-1));
    if PR <= PR_crit
        C = sqrt(gamma * (2/(gamma+1))^((gamma+1)/(gamma-1)));
        m_dot = Area * P_up / sqrt(R * T_up) * C;
    else
        m_dot = Area * P_up / sqrt(R * T_up) * ...
                sqrt(2*gamma/(gamma-1) * (PR^(2/gamma) - PR^((gamma+1)/gamma)));
    end
    m_dot = max(0, m_dot);
end

function T_new = solve_T(T_g, U_tgt, m_tot, V_tank, T_vec, rhoL_vec, rhoV_vec, uL_vec, uV_vec, T_min, T_max)
%#codegen
    T = T_g;
    for k = 1:5
        T = max(T_min, min(T_max, T));
        rL = interp1_lut(T_vec, rhoL_vec, T);
        rV = interp1_lut(T_vec, rhoV_vec, T);
        uL = interp1_lut(T_vec, uL_vec, T);
        uV = interp1_lut(T_vec, uV_vec, T);

        d = 1 - rV / rL;
        if abs(d) < 1e-12; break; end
        ml = max(0, min(m_tot, (m_tot - rV * V_tank) / d));
        mv = m_tot - ml;
        U_c = ml * uL + mv * uV;
        res = U_tgt - U_c;
        if abs(res) < 1.0; break; end

        dT = 0.05;
        Tp = min(T_max, T + dT);
        rLp = interp1_lut(T_vec, rhoL_vec, Tp);
        rVp = interp1_lut(T_vec, rhoV_vec, Tp);
        uLp = interp1_lut(T_vec, uL_vec, Tp);
        uVp = interp1_lut(T_vec, uV_vec, Tp);
        dp = 1 - rVp / rLp;
        if abs(dp) < 1e-12; break; end
        mlp = max(0, min(m_tot, (m_tot - rVp * V_tank) / dp));
        mvp = m_tot - mlp;
        Up = mlp * uLp + mvp * uVp;
        dUdT = (Up - U_c) / dT;
        if abs(dUdT) < 1e-3; break; end

        step = max(-2, min(2, res / dUdT));
        T = T + step;
    end
    T_new = max(T_min, min(T_max, T));
end

== matlab function EReg_Tank_Drain/Servo Actuated Valve/ Valve Gear Conversion ==
  data: servo_angle input; valve_angle output
function valve_angle = fcn(servo_angle)

valve_angle = servo_angle/1.7; % check gear ratio with oscar
%valve_angle = servo_angle;

== matlab function EReg_Tank_Drain/Servo Actuated Valve/ Valve area ==
  data: valve_angle input; valve_area output
function valve_area = fcn(valve_angle)
valve_angle = valve_angle - 5; %Account for first part of rotation where valve doesn't open at all
if valve_angle < 0
    valve_area = 0;
else
    valve_area = 1.1*((5*10^-6)*valve_angle^3 - 0.0006*valve_angle^2 + 0.0278*valve_angle); %calculate normalised valve area
end

== matlab function EReg_Tank_Drain/Servo Actuated Valve/Servo/Signal normalisation ==
  data: u input; y output
function y = fcn(u)
if u < 0
    y = 0;
else 
    if u > 180
        y = 180;
    else
        y = u;
    end
end
